simulink model "dummpy_joint_1"  (R2024b)
settings: Solver=FixedStepAuto  StartTime=0.0  StopTime=10.0  FixedStep=0.001  RelTol=1e-3
libraries: simulink x1
settings Model: Creator=giang  LastModifiedBy=giang

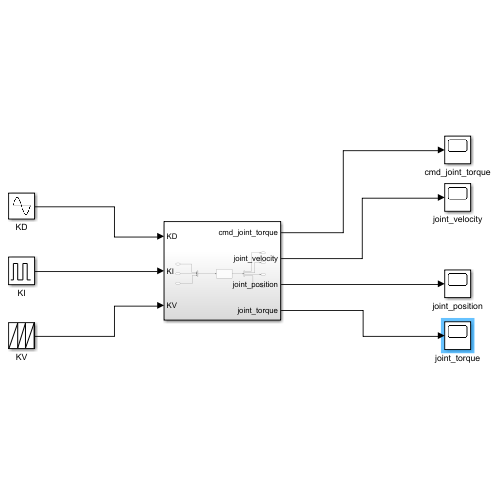
[thumbnail: Simulink's stored preview of the top-level diagram]
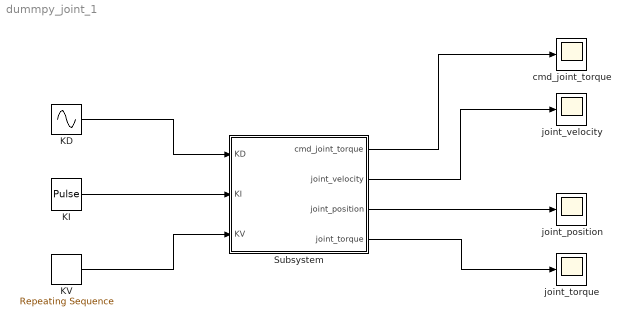
== system dummpy_joint_1 ==
  KD : Sin  Amplitude=[1]  SampleTime=0
  KI : DiscretePulseGenerator  PulseType=Time based  Period=1  PulseWidth=50
  KV : simulink/Sources/Repeating Sequence  rep_seq_t=[0 2]  rep_seq_y=[0 2]
  Subsystem : Subsystem
  cmd_joint_torque : Scope
  joint_position : Scope
  joint_torque : Scope
  joint_velocity : Scope
  wires:
  KD/1 -> Subsystem/1(KD)
  KI/1 -> Subsystem/2(KI)
  KV/1 -> Subsystem/3(KV)
  Subsystem/1(cmd_joint_torque) -> cmd_joint_torque/1
  Subsystem/2(joint_velocity) -> joint_velocity/1
  Subsystem/3(joint_position) -> joint_position/1
  Subsystem/4(joint_torque) -> joint_torque/1

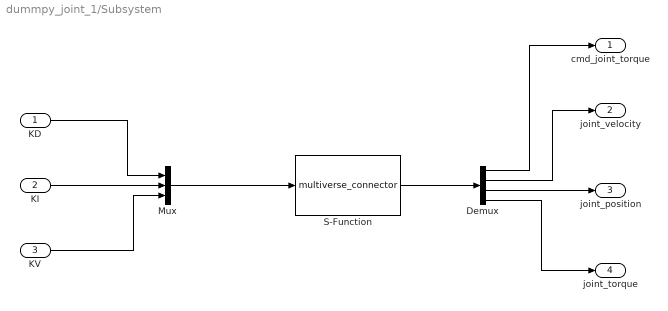
== system dummpy_joint_1/Subsystem ==
  KD : Inport
  KI : Inport  Port=2
  KV : Inport  Port=3
  Demux : Demux
  Mux : Mux  Inputs=3
  S-Function : S-Function  FunctionName=multiverse_connector  Parameters="'tcp://127.0.0.1' '7000' '7593' 'world' 'matlab' '{\"send\": {\"KD\": [\"scalar\"], \"KV\": [\"scalar\"], \"KI\": [\"scalar\"]}, \"receive\": {\"joint_1\": [\"cmd_joint_torque\", \"joint_rvalue\", \"joint_angular_velocity\", \"joint_torque\"]}}'"  SFunctionDeploymentMode=off  EnableBusSupport=off
  cmd_joint_torque : Outport
  joint_velocity : Outport  Port=2
  joint_position : Outport  Port=3
  joint_torque : Outport  Port=4
  wires:
  Mux/1 -> S-Function/1
  S-Function/1 -> Demux/1
  KV/1 -> Mux/3
  KI/1 -> Mux/2
  Demux/4 -> joint_torque/1
  Demux/2 -> joint_velocity/1
  Demux/1 -> cmd_joint_torque/1
  KD/1 -> Mux/1
  Demux/3 -> joint_position/1
